simulink model "ZeroImpactNoZeroCondition"  (R2017a)
settings: Solver=VariableStepAuto  StartTime=0.0  StopTime=25  MaxStep=0.01  RelTol=1e-3
settings Model: Creator=drone  LastModifiedBy=drone

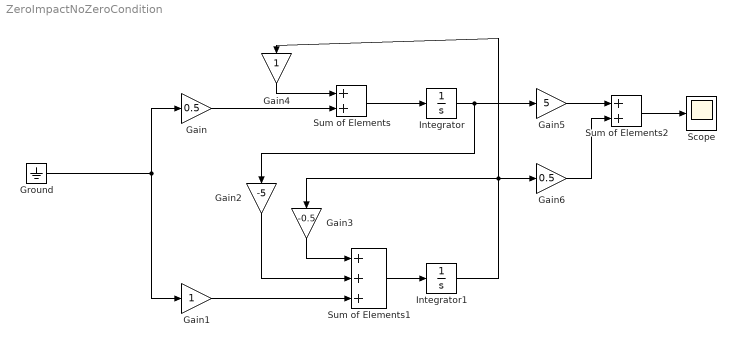
== system ZeroImpactNoZeroCondition ==
  Gain : Gain  Gain=0.5
  Gain1 : Gain
  Gain2 : Gain  Gain=-5
  Gain3 : Gain  Gain=-0.5
  Gain4 : Gain
  Gain5 : Gain  Gain=5
  Gain6 : Gain  Gain=0.5
  Ground : Ground
  Integrator : Integrator  InitialCondition=0.2
  Integrator1 : Integrator  InitialCondition=0.1
  Scope : Scope
  Sum of Elements : Sum  Inputs=2
  Sum of Elements1 : Sum  Inputs=3
  Sum of Elements2 : Sum  Inputs=2
  wires:
  Sum of Elements1/1 -> Integrator1/1
  Gain5/1 -> Sum of Elements2/1
  Ground/1 -> Gain1/1, Gain/1
  Gain4/1 -> Sum of Elements/1
  Sum of Elements/1 -> Integrator/1
  Gain1/1 -> Sum of Elements1/3
  Integrator1/1 -> Gain6/1, Gain3/1, Gain4/1
  Integrator/1 -> Gain2/1, Gain5/1
  Gain6/1 -> Sum of Elements2/2
  Sum of Elements2/1 -> Scope/1
  Gain3/1 -> Sum of Elements1/1
  Gain/1 -> Sum of Elements/2
  Gain2/1 -> Sum of Elements1/2
